simulink model "exp9_"  (R2021b)
settings: Solver=VariableStepAuto  StartTime=0.0  StopTime=100  RelTol=1e-3
undefined symbols (not defined in the file or in its folder): k, k2, k3
libraries: spspowerguiLib x2
settings Model: Creator=amans  LastModifiedBy=amans

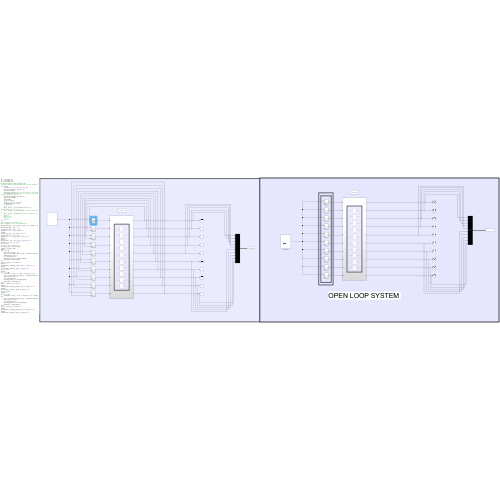
[thumbnail: Simulink's stored preview of the top-level diagram]
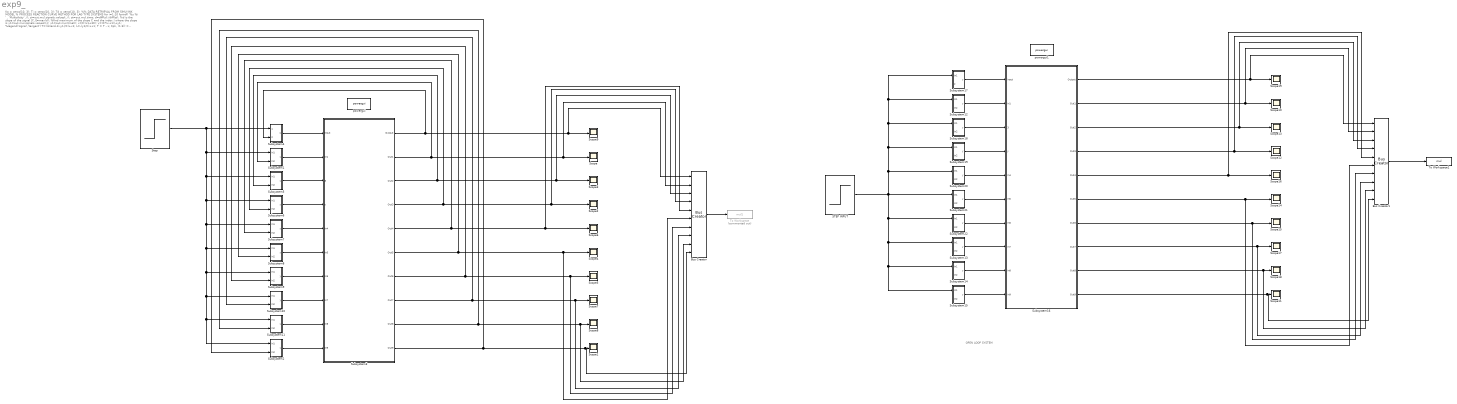
== system exp9_ ==
  note: OPEN LOOP SYSTEM
  note: Kp = zeros(10, 3);
      | Ti = zeros(10, 3);
      | Td = zeros(10, 3);
      | %% DATA RETRIEVAL FROM SIMULINK MODEL
      | % PROCESS REACTION CURVE METHOD FOR LAG TYPE SYSTEMS
      | for i=1:10
      | fprintf( '%s %i\n' , 'Multiplicity' ,i);
      | si=out.mul.signals.values(:,i);
      | st=out.mul.time;
      | d=diff(si)./diff(st); %d is the slope of the signal
      | [C,I]=max(d); %find maximum of the slope C and the index I where the slope is
      | y1=out.mul.signals.values(I,i);
      | x1=out.mul.time(I);
      | x=0:(x1+30);
      | y=(C*(x-x1))+y1;
      | %legend('signal','tangent')
      | T=((si(end-1)-y1)/C)+x1;
      | L=-(y1/C)+x1;
      | T = T - L;
      | Kp(i, (1:3)) = [(T)/L;0.9*T/L;1.2*T/L]; % prooprtional gain for P, Pi, Pid
      | Ti(i, (1:3)) = [-1;L/0.3;2*L]; % time constant for I
      | Td(i, (1:3)) = [0;0;0.5*L]; % time constant for D
      | %hold on
      | %plot(st,si)
      | %plot(x,y);
      | %hold on
      | end
      | %% Dependencies on Multiplicity
      | mul = (1:10); % array for multiplicity
      | scatter(mul,Kp(:, 1)); grid on ; grid minor ; hold on ; % P
      | scatter(mul,Kp(:, 2)); % PI
      | scatter(mul,Kp(:, 3)); % PID
      | legend( 'P' , 'PI' , 'PID' ); hold off ;
      | figure;
      | scatter(mul,Ti(:, 2));hold on ; % PI;
      | scatter(mul,Ti(:, 3)); %PID;
      | legend( 'PI' , 'PID' ); grid on ; grid minor ;
      | hold off ;
      | figure;
      | scatter(mul, Td(:, 3)); grid on ; grid minor ;
      | legend( 'Td vs mul for PID' )
      | %% P CONTROL
      | s = tf( 's' ); H = 1/(s+1.5);
      | settling_Time = zeros(1, 10);
      | oshoot = zeros(1, 10);
      | figure;
      | for i = 1:10
      | controller = Kp(i, 1);
      | cltf = ((controller)*(H^i))/(1 + controller*(H^i));
      | step(cltf); hold on ;
      | A = stepinfo(cltf);
      | settling_Time(i) = A.SettlingTime;
      | oshoot(i) = A.Overshoot;
      | end
      | grid on ; grid minor ; hold off ;
      | figure;
      | scatter(mul, settling_Time); grid on ; grid minor ;
      | figure;
      | scatter(mul, oshoot); grid on ; grid minor ;
      | %% PI control
      | figure;
      | for i = 1:10
      | controller = Kp(i, 2) + Kp(i, 2)/(s*Ti(i, 2));
      | cltf = ((controller)*(H^i))/(1 + controller*(H^i));
      | step(cltf); hold on ;
      | A = stepinfo(cltf);
      | settling_Time(i) = A.SettlingTime;
      | oshoot(i) = A.Overshoot;
      | end
      | grid on ; grid minor ; hold off ;
      | figure;
      | scatter(mul, settling_Time); grid on ; grid minor ;
      | figure;
      | scatter(mul, oshoot); grid on ; grid minor ;
      | %% PID CONTROL
      | figure;
      | for i = 1:10
      | controller = Kp(i, 3)*(1 + 1/(s*Ti(i, 3)) + s*Td(i, 3));
      | cltf = ((controller)*(H^i))/(1 + controller*(H^i));
      | step(cltf); hold on ;
      | A = stepinfo(cltf);
      | settling_Time(i) = A.SettlingTime;
      | oshoot(i) = A.Overshoot;
      | end
      | grid on ; grid minor ; hold off ;
      | figure;
      | scatter(mul, settling_Time); grid on ; grid minor ;
      | figure;
      | scatter(mul, oshoot); grid on ; grid minor ;
  Bus Creator : BusCreator  Inputs=10
  Bus Creator1 : BusCreator  Inputs=10
  STEP INPUT : Step  Time=0  SampleTime=0
  Scope{,1..19} (20 alike) : Scope
  Step : Step  SampleTime=0
  Subsystem1 : Subsystem
  Subsystem10 : Subsystem
  Subsystem11 : Subsystem
  Subsystem12 : Subsystem
  Subsystem13 : Subsystem
  Subsystem14 : Subsystem
  Subsystem15 : Subsystem
  Subsystem16 : Subsystem
  Subsystem17 : Subsystem
  Subsystem18 : Subsystem
  Subsystem19 : Subsystem
  Subsystem2 : Subsystem
  Subsystem20 : Subsystem
  Subsystem21 : Subsystem
  Subsystem22 : Subsystem
  Subsystem3 : Subsystem
  Subsystem4 : Subsystem
  Subsystem5 : Subsystem
  Subsystem6 : Subsystem
  Subsystem7 : Subsystem
  Subsystem8 : Subsystem
  Subsystem9 : Subsystem
  To Workspace : ToWorkspace  Commented=on  VariableName=mul1  SaveFormat=Structure With Time  SampleTime=-1
  To Workspace1 : ToWorkspace  VariableName=mul  SaveFormat=Structure With Time  SampleTime=-1
  powergui : spspowerguiLib/powergui  Priority=1  SimulationMode=Continuous  SampleTime=50e-6  frequency=60  Iterations=50  frequencyindice=60  Pbase=100e6  ErrMax=1e-4  UnitsV=kV  UnitsW=MW  buscounter=0  FunctionMessages=off  echomessages=off  EnableUseOfTLC=off  CurrentSourceSwitches=off  DisableSnubberDevices=off  DisableRonSwitches=off  DisableVfSwitches=off  DisplayEquations=off  AutomaticDiscreteSolvers=off  SolverType=Tustin/Backward Euler (TBE)  Interpol=off  ExternalGateDelay=off  methode=off  Ts=100  x0status=blocks  SPID=on  SwTol=0  HookPort=off  NonlinearTolerance=1e-4  nMaxIteration=100  ContinueOnMaxIteration=off  RestoreLinks=warning  ResistiveCurrentMeasurement=off  Frange=[0:2:500]  Ylog=off  Xlog=on  ShowGrid=off  save=off  variable=ZData  structure=0  ZoomFFT=off  StartTime=0.0  cycles=1  DisplayStyle=1  fundamental=60  FreqAxis=off  MaxFrequency=1000  frequencyindicesteady=1  RmsSteady=1  display=off
  powergui1 : spspowerguiLib/powergui  Priority=1  SimulationMode=Continuous  SampleTime=50e-6  frequency=60  Iterations=50  frequencyindice=60  Pbase=100e6  ErrMax=1e-4  UnitsV=kV  UnitsW=MW  buscounter=0  FunctionMessages=off  echomessages=off  EnableUseOfTLC=off  CurrentSourceSwitches=off  DisableSnubberDevices=off  DisableRonSwitches=off  DisableVfSwitches=off  DisplayEquations=off  AutomaticDiscreteSolvers=off  SolverType=Tustin/Backward Euler (TBE)  Interpol=off  ExternalGateDelay=off  methode=off  Ts=100  x0status=blocks  SPID=on  SwTol=0  HookPort=off  NonlinearTolerance=1e-4  nMaxIteration=100  ContinueOnMaxIteration=off  RestoreLinks=warning  ResistiveCurrentMeasurement=off  Frange=[0:2:500]  Ylog=off  Xlog=on  ShowGrid=off  save=off  variable=ZData  structure=0  ZoomFFT=off  StartTime=0.0  cycles=1  DisplayStyle=1  fundamental=60  FreqAxis=off  MaxFrequency=1000  frequencyindicesteady=1  RmsSteady=1  display=off
  wires:
  Subsystem1/1(y) -> Subsystem3/2(In1)
  Step/1 -> Subsystem9/1(In1), Subsystem10/1(In1), Subsystem2/1(In1), Subsystem11/1(In1), Subsystem8/1(In1), Subsystem7/1(In1), Subsystem6/1(In1), Subsystem5/1(In1), Subsystem1/1(In1), Subsystem4/1(Reference input)
  Subsystem2/1(y) -> Subsystem3/10(In9)
  Subsystem3/10(Out9) -> Bus Creator/10, Scope1/1, Subsystem2/2(In2)
  Subsystem3/2(Out1) -> Subsystem1/2(In2), Scope/1, Bus Creator/2
  Subsystem3/3(Out2) -> Subsystem5/2(In2), Scope3/1, Bus Creator/3
  Subsystem3/5(Out4) -> Subsystem7/2(In2), Scope6/1, Bus Creator/5
  Subsystem3/8(Out7) -> Subsystem10/2(In2), Scope7/1, Bus Creator/8
  Subsystem3/9(Out8) -> Subsystem11/2(In2), Bus Creator/9, Scope8/1
  Subsystem3/1(Output) -> Subsystem4/2(From output), Bus Creator/1, Scope9/1
  Subsystem4/1(To Plant) -> Subsystem3/1(Input)
  Subsystem5/1(y) -> Subsystem3/3(3)
  Subsystem6/1(y) -> Subsystem3/4(y)
  Subsystem7/1(y) -> Subsystem3/5(In4)
  Subsystem8/1(y) -> Subsystem3/6(In5)
  Subsystem3/6(Out5) -> Subsystem8/2(In2), Scope4/1, Bus Creator/6
  Subsystem9/1(y) -> Subsystem3/7(In6)
  Subsystem3/7(Out6) -> Subsystem9/2(In2), Scope5/1, Bus Creator/7
  Subsystem10/1(y) -> Subsystem3/8(In7)
  Subsystem11/1(y) -> Subsystem3/9(In8)
  Bus Creator/1 -> To Workspace/1
  Subsystem3/4(Out3) -> Subsystem6/2(In2), Scope2/1, Bus Creator/4
  Subsystem22/1(y) -> Subsystem16/7(In6)
  Subsystem16/9(Out8) -> Bus Creator1/9, Scope18/1
  Subsystem17/1(y) -> Subsystem16/1(Input)
  Subsystem16/4(Out3) -> Scope12/1, Bus Creator1/4
  Subsystem16/1(Output) -> Bus Creator1/1, Scope19/1
  Subsystem16/7(Out6) -> Scope15/1, Bus Creator1/7
  Subsystem20/1(y) -> Subsystem16/5(In4)
  Subsystem18/1(y) -> Subsystem16/3(3)
  Subsystem12/1(y) -> Subsystem16/2(In1)
  Subsystem16/5(Out4) -> Scope16/1, Bus Creator1/5
  Subsystem15/1(y) -> Subsystem16/10(In9)
  Bus Creator1/1 -> To Workspace1/1
  Subsystem19/1(y) -> Subsystem16/4(y)
  Subsystem21/1(y) -> Subsystem16/6(In5)
  Subsystem16/10(Out9) -> Bus Creator1/10, Scope11/1
  Subsystem16/2(Out1) -> Scope10/1, Bus Creator1/2
  Subsystem16/3(Out2) -> Scope13/1, Bus Creator1/3
  Subsystem13/1(y) -> Subsystem16/8(In7)
  Subsystem14/1(y) -> Subsystem16/9(In8)
  Subsystem16/6(Out5) -> Scope14/1, Bus Creator1/6
  Subsystem16/8(Out7) -> Scope17/1, Bus Creator1/8
  STEP INPUT/1 -> Subsystem17/1(In1), Subsystem12/1(In1), Subsystem18/1(In1), Subsystem19/1(In1), Subsystem20/1(In1), Subsystem22/1(In1), Subsystem13/1(In1), Subsystem15/1(In1), Subsystem14/1(In1), Subsystem21/1(In1)

== system exp9_/Subsystem1 ==
  In1 : Inport
  In2 : Inport  Port=2
  Sum : Sum  Inputs=|+-
  y : Outport
  wires:
  In1/1 -> Sum/1
  In2/1 -> Sum/2
  Sum/1 -> y/1

== system exp9_/Subsystem10 ==
  In1 : Inport
  In2 : Inport  Port=2
  Sum : Sum  Inputs=|+-
  y : Outport
  wires:
  In1/1 -> Sum/1
  In2/1 -> Sum/2
  Sum/1 -> y/1

== system exp9_/Subsystem11 ==
  In1 : Inport
  In2 : Inport  Port=2
  Sum : Sum  Inputs=|+-
  y : Outport
  wires:
  In1/1 -> Sum/1
  In2/1 -> Sum/2
  Sum/1 -> y/1

== system exp9_/Subsystem12 ==
  In1 : Inport
  In2 : Inport  Port=2
  Sum : Sum  Inputs=|+-
  y : Outport
  wires:
  In1/1 -> Sum/1
  In2/1 -> Sum/2
  Sum/1 -> y/1

== system exp9_/Subsystem13 ==
  In1 : Inport
  In2 : Inport  Port=2
  Sum : Sum  Inputs=|+-
  y : Outport
  wires:
  In1/1 -> Sum/1
  In2/1 -> Sum/2
  Sum/1 -> y/1

== system exp9_/Subsystem14 ==
  In1 : Inport
  In2 : Inport  Port=2
  Sum : Sum  Inputs=|+-
  y : Outport
  wires:
  In1/1 -> Sum/1
  In2/1 -> Sum/2
  Sum/1 -> y/1

== system exp9_/Subsystem15 ==
  In1 : Inport
  In2 : Inport  Port=2
  Sum : Sum  Inputs=|+-
  y : Outport
  wires:
  In1/1 -> Sum/1
  In2/1 -> Sum/2
  Sum/1 -> y/1

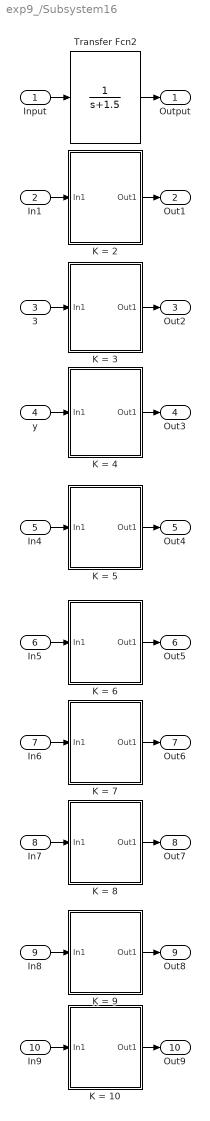
== system exp9_/Subsystem16 ==
  Input : Inport
  In1 : Inport  Port=2
  3 : Inport  Port=3
  y : Inport  Port=4
  In4 : Inport  Port=5
  In5 : Inport  Port=6
  In6 : Inport  Port=7
  In7 : Inport  Port=8
  In8 : Inport  Port=9
  In9 : Inport  Port=10
  K = 10 : Subsystem
  K = 2 : Subsystem
  K = 3 : Subsystem
  K = 4 : Subsystem
  K = 5 : Subsystem
  K = 6 : Subsystem
  K = 7 : Subsystem
  K = 8 : Subsystem
  K = 9 : Subsystem
  Transfer Fcn2 : TransferFcn  Denominator=[1 1.5]
  Output : Outport
  Out1 : Outport  Port=2
  Out2 : Outport  Port=3
  Out3 : Outport  Port=4
  Out4 : Outport  Port=5
  Out5 : Outport  Port=6
  Out6 : Outport  Port=7
  Out7 : Outport  Port=8
  Out8 : Outport  Port=9
  Out9 : Outport  Port=10
  wires:
  K = 8/1(Out1) -> Out7/1
  3/1 -> K = 3/1(In1)
  In9/1 -> K = 10/1(In1)
  K = 6/1(Out1) -> Out5/1
  K = 3/1(Out1) -> Out2/1
  K = 9/1(Out1) -> Out8/1
  K = 2/1(Out1) -> Out1/1
  In8/1 -> K = 9/1(In1)
  K = 10/1(Out1) -> Out9/1
  In6/1 -> K = 7/1(In1)
  In4/1 -> K = 5/1(In1)
  In7/1 -> K = 8/1(In1)
  K = 4/1(Out1) -> Out3/1
  y/1 -> K = 4/1(In1)
  K = 7/1(Out1) -> Out6/1
  In5/1 -> K = 6/1(In1)
  In1/1 -> K = 2/1(In1)
  K = 5/1(Out1) -> Out4/1
  Input/1 -> Transfer Fcn2/1
  Transfer Fcn2/1 -> Output/1

== system exp9_/Subsystem17 ==
  In1 : Inport
  Output : Inport  Port=2
  Sum : Sum  Inputs=|+-
  y : Outport
  wires:
  In1/1 -> Sum/1
  Output/1 -> Sum/2
  Sum/1 -> y/1

== system exp9_/Subsystem18 ==
  In1 : Inport
  In2 : Inport  Port=2
  Sum : Sum  Inputs=|+-
  y : Outport
  wires:
  In1/1 -> Sum/1
  In2/1 -> Sum/2
  Sum/1 -> y/1

== system exp9_/Subsystem19 ==
  In1 : Inport
  In2 : Inport  Port=2
  Sum : Sum  Inputs=|+-
  y : Outport
  wires:
  In1/1 -> Sum/1
  In2/1 -> Sum/2
  Sum/1 -> y/1

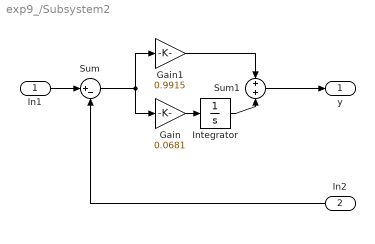
== system exp9_/Subsystem2 ==
  In1 : Inport
  In2 : Inport  Port=2
  Gain : Gain  Gain=0.0681
  Gain1 : Gain  Gain=0.9915
  Integrator : Integrator
  Sum : Sum  Inputs=|+-
  Sum1 : Sum  Inputs=+|+
  y : Outport
  wires:
  In1/1 -> Sum/1
  In2/1 -> Sum/2
  Gain/1 -> Integrator/1
  Sum/1 -> Gain1/1, Gain/1
  Sum1/1 -> y/1
  Integrator/1 -> Sum1/2
  Gain1/1 -> Sum1/1

== system exp9_/Subsystem20 ==
  In1 : Inport
  In2 : Inport  Port=2
  Sum : Sum  Inputs=|+-
  y : Outport
  wires:
  In1/1 -> Sum/1
  In2/1 -> Sum/2
  Sum/1 -> y/1

== system exp9_/Subsystem21 ==
  In1 : Inport
  In2 : Inport  Port=2
  Sum : Sum  Inputs=|+-
  y : Outport
  wires:
  In1/1 -> Sum/1
  In2/1 -> Sum/2
  Sum/1 -> y/1

== system exp9_/Subsystem22 ==
  In1 : Inport
  In2 : Inport  Port=2
  Sum : Sum  Inputs=|+-
  y : Outport
  wires:
  In1/1 -> Sum/1
  In2/1 -> Sum/2
  Sum/1 -> y/1

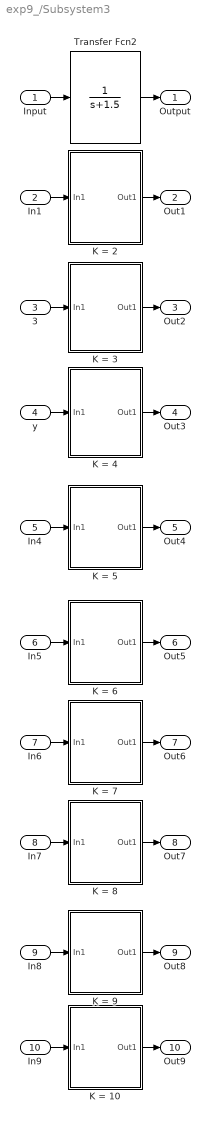
== system exp9_/Subsystem3 ==
  Input : Inport
  In1 : Inport  Port=2
  3 : Inport  Port=3
  y : Inport  Port=4
  In4 : Inport  Port=5
  In5 : Inport  Port=6
  In6 : Inport  Port=7
  In7 : Inport  Port=8
  In8 : Inport  Port=9
  In9 : Inport  Port=10
  K = 10 : Subsystem
  K = 2 : Subsystem
  K = 3 : Subsystem
  K = 4 : Subsystem
  K = 5 : Subsystem
  K = 6 : Subsystem
  K = 7 : Subsystem
  K = 8 : Subsystem
  K = 9 : Subsystem
  Transfer Fcn2 : TransferFcn  Denominator=[1 1.5]
  Output : Outport
  Out1 : Outport  Port=2
  Out2 : Outport  Port=3
  Out3 : Outport  Port=4
  Out4 : Outport  Port=5
  Out5 : Outport  Port=6
  Out6 : Outport  Port=7
  Out7 : Outport  Port=8
  Out8 : Outport  Port=9
  Out9 : Outport  Port=10
  wires:
  K = 8/1(Out1) -> Out7/1
  3/1 -> K = 3/1(In1)
  In9/1 -> K = 10/1(In1)
  K = 6/1(Out1) -> Out5/1
  K = 3/1(Out1) -> Out2/1
  K = 9/1(Out1) -> Out8/1
  K = 2/1(Out1) -> Out1/1
  In8/1 -> K = 9/1(In1)
  K = 10/1(Out1) -> Out9/1
  In6/1 -> K = 7/1(In1)
  In4/1 -> K = 5/1(In1)
  In7/1 -> K = 8/1(In1)
  K = 4/1(Out1) -> Out3/1
  y/1 -> K = 4/1(In1)
  K = 7/1(Out1) -> Out6/1
  In5/1 -> K = 6/1(In1)
  In1/1 -> K = 2/1(In1)
  K = 5/1(Out1) -> Out4/1
  Input/1 -> Transfer Fcn2/1
  Transfer Fcn2/1 -> Output/1

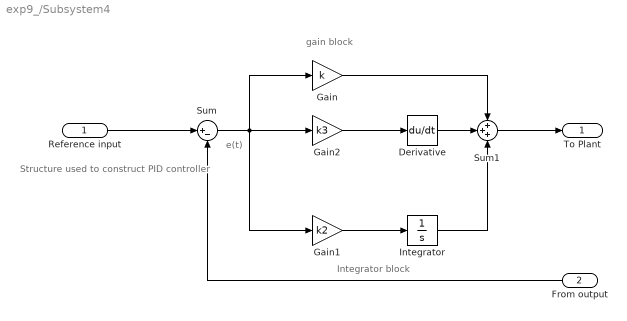
== system exp9_/Subsystem4 ==
  note: Integrator block
  note: Structure used to construct PID controller
  note: gain block
  note: e(t)
  Reference input : Inport
  From output : Inport  Port=2
  Derivative : Derivative
  Gain : Gain  Gain=k
  Gain1 : Gain  Gain=k2
  Gain2 : Gain  Gain=k3
  Integrator : Integrator
  Sum : Sum  Inputs=|+-
  Sum1 : Sum  Inputs=+++
  To Plant : Outport
  wires:
  Reference input/1 -> Sum/1
  From output/1 -> Sum/2
  Sum/1 -> Gain2/1, Gain/1, Gain1/1
  Integrator/1 -> Sum1/3
  Sum1/1 -> To Plant/1
  Gain/1 -> Sum1/1
  Gain1/1 -> Integrator/1
  Derivative/1 -> Sum1/2
  Gain2/1 -> Derivative/1

== system exp9_/Subsystem5 ==
  In1 : Inport
  In2 : Inport  Port=2
  Sum : Sum  Inputs=|+-
  y : Outport
  wires:
  In1/1 -> Sum/1
  In2/1 -> Sum/2
  Sum/1 -> y/1

== system exp9_/Subsystem6 ==
  In1 : Inport
  In2 : Inport  Port=2
  Sum : Sum  Inputs=|+-
  y : Outport
  wires:
  In1/1 -> Sum/1
  In2/1 -> Sum/2
  Sum/1 -> y/1

== system exp9_/Subsystem7 ==
  In1 : Inport
  In2 : Inport  Port=2
  Sum : Sum  Inputs=|+-
  y : Outport
  wires:
  In1/1 -> Sum/1
  In2/1 -> Sum/2
  Sum/1 -> y/1

== system exp9_/Subsystem8 ==
  In1 : Inport
  In2 : Inport  Port=2
  Sum : Sum  Inputs=|+-
  y : Outport
  wires:
  In1/1 -> Sum/1
  In2/1 -> Sum/2
  Sum/1 -> y/1

== system exp9_/Subsystem9 ==
  In1 : Inport
  In2 : Inport  Port=2
  Sum : Sum  Inputs=|+-
  y : Outport
  wires:
  In1/1 -> Sum/1
  In2/1 -> Sum/2
  Sum/1 -> y/1

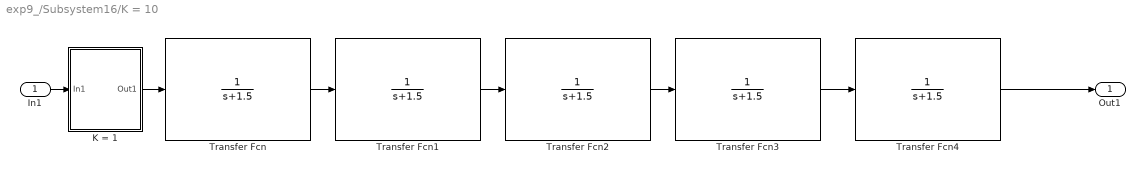
== system exp9_/Subsystem16/K = 10 ==
  In1 : Inport
  K = 1 : Subsystem
  Transfer Fcn{,1..4} (5 alike) : TransferFcn  Denominator=[1 1.5]
  Out1 : Outport
  wires:
  K = 1/1(Out1) -> Transfer Fcn/1
  In1/1 -> K = 1/1(In1)
  Transfer Fcn/1 -> Transfer Fcn1/1
  Transfer Fcn1/1 -> Transfer Fcn2/1
  Transfer Fcn2/1 -> Transfer Fcn3/1
  Transfer Fcn3/1 -> Transfer Fcn4/1
  Transfer Fcn4/1 -> Out1/1

== system exp9_/Subsystem16/K = 2 ==
  In1 : Inport
  Transfer Fcn2 : TransferFcn  Denominator=[1 1.5]
  Transfer Fcn3 : TransferFcn  Denominator=[1 1.5]
  Out1 : Outport
  wires:
  Transfer Fcn2/1 -> Transfer Fcn3/1
  In1/1 -> Transfer Fcn2/1
  Transfer Fcn3/1 -> Out1/1

== system exp9_/Subsystem16/K = 3 ==
  In1 : Inport
  K = 1 : Subsystem
  Transfer Fcn2 : TransferFcn  Denominator=[1 1.5]
  Out1 : Outport
  wires:
  K = 1/1(Out1) -> Transfer Fcn2/1
  Transfer Fcn2/1 -> Out1/1
  In1/1 -> K = 1/1(In1)

== system exp9_/Subsystem16/K = 4 ==
  In1 : Inport
  K = 1 : Subsystem
  Transfer Fcn2 : TransferFcn  Denominator=[1 1.5]
  Out1 : Outport
  wires:
  K = 1/1(Out1) -> Transfer Fcn2/1
  Transfer Fcn2/1 -> Out1/1
  In1/1 -> K = 1/1(In1)

== system exp9_/Subsystem16/K = 5 ==
  In1 : Inport
  K = 1 : Subsystem
  Transfer Fcn : TransferFcn  Denominator=[1 1.5]
  Out1 : Outport
  wires:
  K = 1/1(Out1) -> Transfer Fcn/1
  In1/1 -> K = 1/1(In1)
  Transfer Fcn/1 -> Out1/1

== system exp9_/Subsystem16/K = 6 ==
  In1 : Inport
  K = 1 : Subsystem
  Transfer Fcn : TransferFcn  Denominator=[1 1.5]
  Out1 : Outport
  wires:
  Transfer Fcn/1 -> Out1/1
  K = 1/1(Out1) -> Transfer Fcn/1
  In1/1 -> K = 1/1(In1)

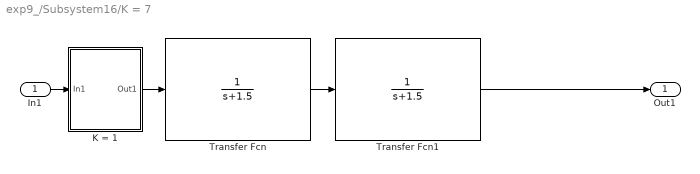
== system exp9_/Subsystem16/K = 7 ==
  In1 : Inport
  K = 1 : Subsystem
  Transfer Fcn : TransferFcn  Denominator=[1 1.5]
  Transfer Fcn1 : TransferFcn  Denominator=[1 1.5]
  Out1 : Outport
  wires:
  K = 1/1(Out1) -> Transfer Fcn/1
  In1/1 -> K = 1/1(In1)
  Transfer Fcn/1 -> Transfer Fcn1/1
  Transfer Fcn1/1 -> Out1/1

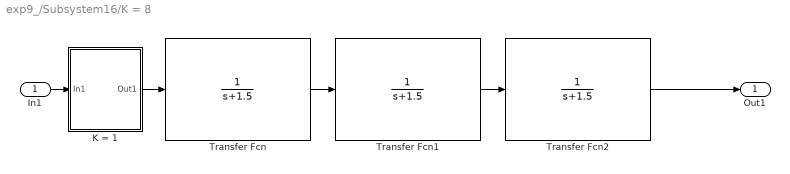
== system exp9_/Subsystem16/K = 8 ==
  In1 : Inport
  K = 1 : Subsystem
  Transfer Fcn : TransferFcn  Denominator=[1 1.5]
  Transfer Fcn1 : TransferFcn  Denominator=[1 1.5]
  Transfer Fcn2 : TransferFcn  Denominator=[1 1.5]
  Out1 : Outport
  wires:
  K = 1/1(Out1) -> Transfer Fcn/1
  In1/1 -> K = 1/1(In1)
  Transfer Fcn/1 -> Transfer Fcn1/1
  Transfer Fcn1/1 -> Transfer Fcn2/1
  Transfer Fcn2/1 -> Out1/1

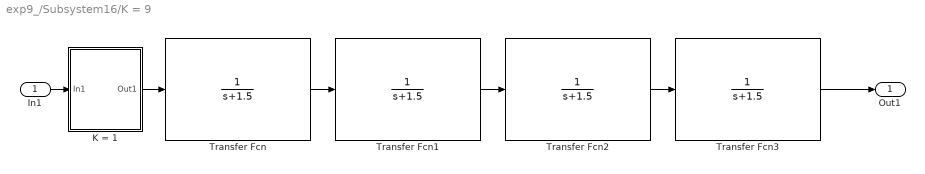
== system exp9_/Subsystem16/K = 9 ==
  In1 : Inport
  K = 1 : Subsystem
  Transfer Fcn{,1..3} (4 alike) : TransferFcn  Denominator=[1 1.5]
  Out1 : Outport
  wires:
  K = 1/1(Out1) -> Transfer Fcn/1
  In1/1 -> K = 1/1(In1)
  Transfer Fcn/1 -> Transfer Fcn1/1
  Transfer Fcn1/1 -> Transfer Fcn2/1
  Transfer Fcn2/1 -> Transfer Fcn3/1
  Transfer Fcn3/1 -> Out1/1

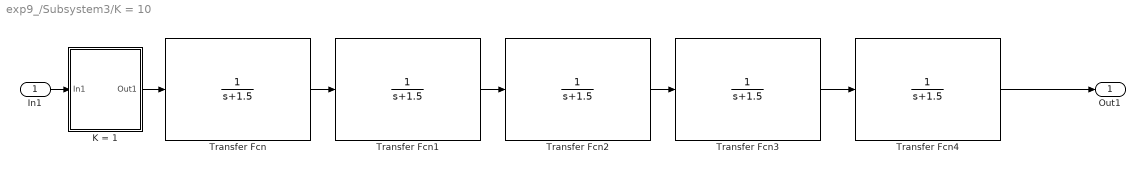
== system exp9_/Subsystem3/K = 10 ==
  In1 : Inport
  K = 1 : Subsystem
  Transfer Fcn{,1..4} (5 alike) : TransferFcn  Denominator=[1 1.5]
  Out1 : Outport
  wires:
  K = 1/1(Out1) -> Transfer Fcn/1
  In1/1 -> K = 1/1(In1)
  Transfer Fcn/1 -> Transfer Fcn1/1
  Transfer Fcn1/1 -> Transfer Fcn2/1
  Transfer Fcn2/1 -> Transfer Fcn3/1
  Transfer Fcn3/1 -> Transfer Fcn4/1
  Transfer Fcn4/1 -> Out1/1

== system exp9_/Subsystem3/K = 2 ==
  In1 : Inport
  Transfer Fcn2 : TransferFcn  Denominator=[1 1.5]
  Transfer Fcn3 : TransferFcn  Denominator=[1 1.5]
  Out1 : Outport
  wires:
  Transfer Fcn2/1 -> Transfer Fcn3/1
  In1/1 -> Transfer Fcn2/1
  Transfer Fcn3/1 -> Out1/1

== system exp9_/Subsystem3/K = 3 ==
  In1 : Inport
  K = 1 : Subsystem
  Transfer Fcn2 : TransferFcn  Denominator=[1 1.5]
  Out1 : Outport
  wires:
  K = 1/1(Out1) -> Transfer Fcn2/1
  Transfer Fcn2/1 -> Out1/1
  In1/1 -> K = 1/1(In1)

== system exp9_/Subsystem3/K = 4 ==
  In1 : Inport
  K = 1 : Subsystem
  Transfer Fcn2 : TransferFcn  Denominator=[1 1.5]
  Out1 : Outport
  wires:
  K = 1/1(Out1) -> Transfer Fcn2/1
  Transfer Fcn2/1 -> Out1/1
  In1/1 -> K = 1/1(In1)

== system exp9_/Subsystem3/K = 5 ==
  In1 : Inport
  K = 1 : Subsystem
  Transfer Fcn : TransferFcn  Denominator=[1 1.5]
  Out1 : Outport
  wires:
  K = 1/1(Out1) -> Transfer Fcn/1
  In1/1 -> K = 1/1(In1)
  Transfer Fcn/1 -> Out1/1

== system exp9_/Subsystem3/K = 6 ==
  In1 : Inport
  K = 1 : Subsystem
  Transfer Fcn : TransferFcn  Denominator=[1 1.5]
  Out1 : Outport
  wires:
  Transfer Fcn/1 -> Out1/1
  K = 1/1(Out1) -> Transfer Fcn/1
  In1/1 -> K = 1/1(In1)

== system exp9_/Subsystem3/K = 7 ==
  In1 : Inport
  K = 1 : Subsystem
  Transfer Fcn : TransferFcn  Denominator=[1 1.5]
  Transfer Fcn1 : TransferFcn  Denominator=[1 1.5]
  Out1 : Outport
  wires:
  K = 1/1(Out1) -> Transfer Fcn/1
  In1/1 -> K = 1/1(In1)
  Transfer Fcn/1 -> Transfer Fcn1/1
  Transfer Fcn1/1 -> Out1/1

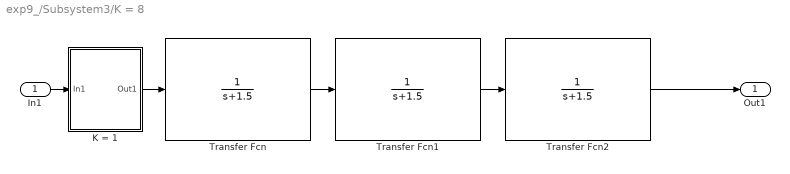
== system exp9_/Subsystem3/K = 8 ==
  In1 : Inport
  K = 1 : Subsystem
  Transfer Fcn : TransferFcn  Denominator=[1 1.5]
  Transfer Fcn1 : TransferFcn  Denominator=[1 1.5]
  Transfer Fcn2 : TransferFcn  Denominator=[1 1.5]
  Out1 : Outport
  wires:
  K = 1/1(Out1) -> Transfer Fcn/1
  In1/1 -> K = 1/1(In1)
  Transfer Fcn/1 -> Transfer Fcn1/1
  Transfer Fcn1/1 -> Transfer Fcn2/1
  Transfer Fcn2/1 -> Out1/1

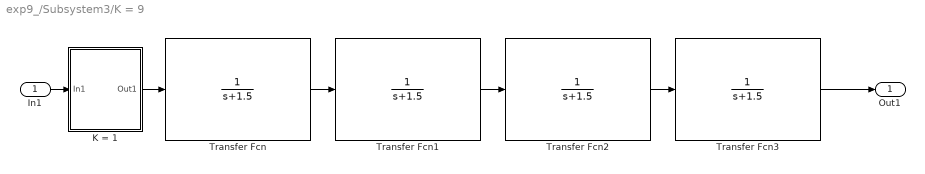
== system exp9_/Subsystem3/K = 9 ==
  In1 : Inport
  K = 1 : Subsystem
  Transfer Fcn{,1..3} (4 alike) : TransferFcn  Denominator=[1 1.5]
  Out1 : Outport
  wires:
  K = 1/1(Out1) -> Transfer Fcn/1
  In1/1 -> K = 1/1(In1)
  Transfer Fcn/1 -> Transfer Fcn1/1
  Transfer Fcn1/1 -> Transfer Fcn2/1
  Transfer Fcn2/1 -> Transfer Fcn3/1
  Transfer Fcn3/1 -> Out1/1

== system exp9_/Subsystem16/K = 10/K = 1 ==
  In1 : Inport
  K = 1 : Subsystem
  Transfer Fcn : TransferFcn  Denominator=[1 1.5]
  Out1 : Outport
  wires:
  K = 1/1(Out1) -> Transfer Fcn/1
  In1/1 -> K = 1/1(In1)
  Transfer Fcn/1 -> Out1/1

== system exp9_/Subsystem16/K = 3/K = 1 ==
  In1 : Inport
  Transfer Fcn2 : TransferFcn  Denominator=[1 1.5]
  Transfer Fcn3 : TransferFcn  Denominator=[1 1.5]
  Out1 : Outport
  wires:
  Transfer Fcn2/1 -> Transfer Fcn3/1
  In1/1 -> Transfer Fcn2/1
  Transfer Fcn3/1 -> Out1/1

== system exp9_/Subsystem16/K = 4/K = 1 ==
  In1 : Inport
  Transfer Fcn2 : TransferFcn  Denominator=[1 1.5]
  Transfer Fcn3 : TransferFcn  Denominator=[1 1.5]
  Out1 : Outport
  wires:
  Transfer Fcn2/1 -> Transfer Fcn3/1
  In1/1 -> Transfer Fcn2/1
  Transfer Fcn3/1 -> Out1/1

== system exp9_/Subsystem16/K = 5/K = 1 ==
  In1 : Inport
  K = 1 : Subsystem
  Transfer Fcn2 : TransferFcn  Denominator=[1 1.5]
  Out1 : Outport
  wires:
  K = 1/1(Out1) -> Transfer Fcn2/1
  Transfer Fcn2/1 -> Out1/1
  In1/1 -> K = 1/1(In1)

== system exp9_/Subsystem16/K = 6/K = 1 ==
  In1 : Inport
  K = 1 : Subsystem
  Transfer Fcn : TransferFcn  Denominator=[1 1.5]
  Out1 : Outport
  wires:
  K = 1/1(Out1) -> Transfer Fcn/1
  In1/1 -> K = 1/1(In1)
  Transfer Fcn/1 -> Out1/1

== system exp9_/Subsystem16/K = 7/K = 1 ==
  In1 : Inport
  K = 1 : Subsystem
  Transfer Fcn : TransferFcn  Denominator=[1 1.5]
  Out1 : Outport
  wires:
  K = 1/1(Out1) -> Transfer Fcn/1
  In1/1 -> K = 1/1(In1)
  Transfer Fcn/1 -> Out1/1

== system exp9_/Subsystem16/K = 8/K = 1 ==
  In1 : Inport
  K = 1 : Subsystem
  Transfer Fcn : TransferFcn  Denominator=[1 1.5]
  Out1 : Outport
  wires:
  K = 1/1(Out1) -> Transfer Fcn/1
  In1/1 -> K = 1/1(In1)
  Transfer Fcn/1 -> Out1/1

== system exp9_/Subsystem16/K = 9/K = 1 ==
  In1 : Inport
  K = 1 : Subsystem
  Transfer Fcn : TransferFcn  Denominator=[1 1.5]
  Out1 : Outport
  wires:
  K = 1/1(Out1) -> Transfer Fcn/1
  In1/1 -> K = 1/1(In1)
  Transfer Fcn/1 -> Out1/1

== system exp9_/Subsystem3/K = 10/K = 1 ==
  In1 : Inport
  K = 1 : Subsystem
  Transfer Fcn : TransferFcn  Denominator=[1 1.5]
  Out1 : Outport
  wires:
  K = 1/1(Out1) -> Transfer Fcn/1
  In1/1 -> K = 1/1(In1)
  Transfer Fcn/1 -> Out1/1

== system exp9_/Subsystem3/K = 3/K = 1 ==
  In1 : Inport
  Transfer Fcn2 : TransferFcn  Denominator=[1 1.5]
  Transfer Fcn3 : TransferFcn  Denominator=[1 1.5]
  Out1 : Outport
  wires:
  Transfer Fcn2/1 -> Transfer Fcn3/1
  In1/1 -> Transfer Fcn2/1
  Transfer Fcn3/1 -> Out1/1

== system exp9_/Subsystem3/K = 4/K = 1 ==
  In1 : Inport
  Transfer Fcn2 : TransferFcn  Denominator=[1 1.5]
  Transfer Fcn3 : TransferFcn  Denominator=[1 1.5]
  Out1 : Outport
  wires:
  Transfer Fcn2/1 -> Transfer Fcn3/1
  In1/1 -> Transfer Fcn2/1
  Transfer Fcn3/1 -> Out1/1

== system exp9_/Subsystem3/K = 5/K = 1 ==
  In1 : Inport
  K = 1 : Subsystem
  Transfer Fcn2 : TransferFcn  Denominator=[1 1.5]
  Out1 : Outport
  wires:
  K = 1/1(Out1) -> Transfer Fcn2/1
  Transfer Fcn2/1 -> Out1/1
  In1/1 -> K = 1/1(In1)

== system exp9_/Subsystem3/K = 6/K = 1 ==
  In1 : Inport
  K = 1 : Subsystem
  Transfer Fcn : TransferFcn  Denominator=[1 1.5]
  Out1 : Outport
  wires:
  K = 1/1(Out1) -> Transfer Fcn/1
  In1/1 -> K = 1/1(In1)
  Transfer Fcn/1 -> Out1/1

== system exp9_/Subsystem3/K = 7/K = 1 ==
  In1 : Inport
  K = 1 : Subsystem
  Transfer Fcn : TransferFcn  Denominator=[1 1.5]
  Out1 : Outport
  wires:
  K = 1/1(Out1) -> Transfer Fcn/1
  In1/1 -> K = 1/1(In1)
  Transfer Fcn/1 -> Out1/1

== system exp9_/Subsystem3/K = 8/K = 1 ==
  In1 : Inport
  K = 1 : Subsystem
  Transfer Fcn : TransferFcn  Denominator=[1 1.5]
  Out1 : Outport
  wires:
  K = 1/1(Out1) -> Transfer Fcn/1
  In1/1 -> K = 1/1(In1)
  Transfer Fcn/1 -> Out1/1

== system exp9_/Subsystem3/K = 9/K = 1 ==
  In1 : Inport
  K = 1 : Subsystem
  Transfer Fcn : TransferFcn  Denominator=[1 1.5]
  Out1 : Outport
  wires:
  K = 1/1(Out1) -> Transfer Fcn/1
  In1/1 -> K = 1/1(In1)
  Transfer Fcn/1 -> Out1/1

== system exp9_/Subsystem16/K = 10/K = 1/K = 1 ==
  In1 : Inport
  K = 1 : Subsystem
  Transfer Fcn2 : TransferFcn  Denominator=[1 1.5]
  Out1 : Outport
  wires:
  K = 1/1(Out1) -> Transfer Fcn2/1
  Transfer Fcn2/1 -> Out1/1
  In1/1 -> K = 1/1(In1)

== system exp9_/Subsystem16/K = 5/K = 1/K = 1 ==
  In1 : Inport
  Transfer Fcn2 : TransferFcn  Denominator=[1 1.5]
  Transfer Fcn3 : TransferFcn  Denominator=[1 1.5]
  Out1 : Outport
  wires:
  Transfer Fcn2/1 -> Transfer Fcn3/1
  In1/1 -> Transfer Fcn2/1
  Transfer Fcn3/1 -> Out1/1

== system exp9_/Subsystem16/K = 6/K = 1/K = 1 ==
  In1 : Inport
  K = 1 : Subsystem
  Transfer Fcn2 : TransferFcn  Denominator=[1 1.5]
  Out1 : Outport
  wires:
  K = 1/1(Out1) -> Transfer Fcn2/1
  Transfer Fcn2/1 -> Out1/1
  In1/1 -> K = 1/1(In1)

== system exp9_/Subsystem16/K = 7/K = 1/K = 1 ==
  In1 : Inport
  K = 1 : Subsystem
  Transfer Fcn2 : TransferFcn  Denominator=[1 1.5]
  Out1 : Outport
  wires:
  K = 1/1(Out1) -> Transfer Fcn2/1
  Transfer Fcn2/1 -> Out1/1
  In1/1 -> K = 1/1(In1)

== system exp9_/Subsystem16/K = 8/K = 1/K = 1 ==
  In1 : Inport
  K = 1 : Subsystem
  Transfer Fcn2 : TransferFcn  Denominator=[1 1.5]
  Out1 : Outport
  wires:
  K = 1/1(Out1) -> Transfer Fcn2/1
  Transfer Fcn2/1 -> Out1/1
  In1/1 -> K = 1/1(In1)

== system exp9_/Subsystem16/K = 9/K = 1/K = 1 ==
  In1 : Inport
  K = 1 : Subsystem
  Transfer Fcn2 : TransferFcn  Denominator=[1 1.5]
  Out1 : Outport
  wires:
  K = 1/1(Out1) -> Transfer Fcn2/1
  Transfer Fcn2/1 -> Out1/1
  In1/1 -> K = 1/1(In1)

== system exp9_/Subsystem3/K = 10/K = 1/K = 1 ==
  In1 : Inport
  K = 1 : Subsystem
  Transfer Fcn2 : TransferFcn  Denominator=[1 1.5]
  Out1 : Outport
  wires:
  K = 1/1(Out1) -> Transfer Fcn2/1
  Transfer Fcn2/1 -> Out1/1
  In1/1 -> K = 1/1(In1)

== system exp9_/Subsystem3/K = 5/K = 1/K = 1 ==
  In1 : Inport
  Transfer Fcn2 : TransferFcn  Denominator=[1 1.5]
  Transfer Fcn3 : TransferFcn  Denominator=[1 1.5]
  Out1 : Outport
  wires:
  Transfer Fcn2/1 -> Transfer Fcn3/1
  In1/1 -> Transfer Fcn2/1
  Transfer Fcn3/1 -> Out1/1

== system exp9_/Subsystem3/K = 6/K = 1/K = 1 ==
  In1 : Inport
  K = 1 : Subsystem
  Transfer Fcn2 : TransferFcn  Denominator=[1 1.5]
  Out1 : Outport
  wires:
  K = 1/1(Out1) -> Transfer Fcn2/1
  Transfer Fcn2/1 -> Out1/1
  In1/1 -> K = 1/1(In1)

== system exp9_/Subsystem3/K = 7/K = 1/K = 1 ==
  In1 : Inport
  K = 1 : Subsystem
  Transfer Fcn2 : TransferFcn  Denominator=[1 1.5]
  Out1 : Outport
  wires:
  K = 1/1(Out1) -> Transfer Fcn2/1
  Transfer Fcn2/1 -> Out1/1
  In1/1 -> K = 1/1(In1)

== system exp9_/Subsystem3/K = 8/K = 1/K = 1 ==
  In1 : Inport
  K = 1 : Subsystem
  Transfer Fcn2 : TransferFcn  Denominator=[1 1.5]
  Out1 : Outport
  wires:
  K = 1/1(Out1) -> Transfer Fcn2/1
  Transfer Fcn2/1 -> Out1/1
  In1/1 -> K = 1/1(In1)

== system exp9_/Subsystem3/K = 9/K = 1/K = 1 ==
  In1 : Inport
  K = 1 : Subsystem
  Transfer Fcn2 : TransferFcn  Denominator=[1 1.5]
  Out1 : Outport
  wires:
  K = 1/1(Out1) -> Transfer Fcn2/1
  Transfer Fcn2/1 -> Out1/1
  In1/1 -> K = 1/1(In1)

== system exp9_/Subsystem16/K = 10/K = 1/K = 1/K = 1 ==
  In1 : Inport
  Transfer Fcn2 : TransferFcn  Denominator=[1 1.5]
  Transfer Fcn3 : TransferFcn  Denominator=[1 1.5]
  Out1 : Outport
  wires:
  Transfer Fcn2/1 -> Transfer Fcn3/1
  In1/1 -> Transfer Fcn2/1
  Transfer Fcn3/1 -> Out1/1

== system exp9_/Subsystem16/K = 6/K = 1/K = 1/K = 1 ==
  In1 : Inport
  Transfer Fcn2 : TransferFcn  Denominator=[1 1.5]
  Transfer Fcn3 : TransferFcn  Denominator=[1 1.5]
  Out1 : Outport
  wires:
  Transfer Fcn2/1 -> Transfer Fcn3/1
  In1/1 -> Transfer Fcn2/1
  Transfer Fcn3/1 -> Out1/1

== system exp9_/Subsystem16/K = 7/K = 1/K = 1/K = 1 ==
  In1 : Inport
  Transfer Fcn2 : TransferFcn  Denominator=[1 1.5]
  Transfer Fcn3 : TransferFcn  Denominator=[1 1.5]
  Out1 : Outport
  wires:
  Transfer Fcn2/1 -> Transfer Fcn3/1
  In1/1 -> Transfer Fcn2/1
  Transfer Fcn3/1 -> Out1/1

== system exp9_/Subsystem16/K = 8/K = 1/K = 1/K = 1 ==
  In1 : Inport
  Transfer Fcn2 : TransferFcn  Denominator=[1 1.5]
  Transfer Fcn3 : TransferFcn  Denominator=[1 1.5]
  Out1 : Outport
  wires:
  Transfer Fcn2/1 -> Transfer Fcn3/1
  In1/1 -> Transfer Fcn2/1
  Transfer Fcn3/1 -> Out1/1

== system exp9_/Subsystem16/K = 9/K = 1/K = 1/K = 1 ==
  In1 : Inport
  Transfer Fcn2 : TransferFcn  Denominator=[1 1.5]
  Transfer Fcn3 : TransferFcn  Denominator=[1 1.5]
  Out1 : Outport
  wires:
  Transfer Fcn2/1 -> Transfer Fcn3/1
  In1/1 -> Transfer Fcn2/1
  Transfer Fcn3/1 -> Out1/1

== system exp9_/Subsystem3/K = 10/K = 1/K = 1/K = 1 ==
  In1 : Inport
  Transfer Fcn2 : TransferFcn  Denominator=[1 1.5]
  Transfer Fcn3 : TransferFcn  Denominator=[1 1.5]
  Out1 : Outport
  wires:
  Transfer Fcn2/1 -> Transfer Fcn3/1
  In1/1 -> Transfer Fcn2/1
  Transfer Fcn3/1 -> Out1/1

== system exp9_/Subsystem3/K = 6/K = 1/K = 1/K = 1 ==
  In1 : Inport
  Transfer Fcn2 : TransferFcn  Denominator=[1 1.5]
  Transfer Fcn3 : TransferFcn  Denominator=[1 1.5]
  Out1 : Outport
  wires:
  Transfer Fcn2/1 -> Transfer Fcn3/1
  In1/1 -> Transfer Fcn2/1
  Transfer Fcn3/1 -> Out1/1

== system exp9_/Subsystem3/K = 7/K = 1/K = 1/K = 1 ==
  In1 : Inport
  Transfer Fcn2 : TransferFcn  Denominator=[1 1.5]
  Transfer Fcn3 : TransferFcn  Denominator=[1 1.5]
  Out1 : Outport
  wires:
  Transfer Fcn2/1 -> Transfer Fcn3/1
  In1/1 -> Transfer Fcn2/1
  Transfer Fcn3/1 -> Out1/1

== system exp9_/Subsystem3/K = 8/K = 1/K = 1/K = 1 ==
  In1 : Inport
  Transfer Fcn2 : TransferFcn  Denominator=[1 1.5]
  Transfer Fcn3 : TransferFcn  Denominator=[1 1.5]
  Out1 : Outport
  wires:
  Transfer Fcn2/1 -> Transfer Fcn3/1
  In1/1 -> Transfer Fcn2/1
  Transfer Fcn3/1 -> Out1/1

== system exp9_/Subsystem3/K = 9/K = 1/K = 1/K = 1 ==
  In1 : Inport
  Transfer Fcn2 : TransferFcn  Denominator=[1 1.5]
  Transfer Fcn3 : TransferFcn  Denominator=[1 1.5]
  Out1 : Outport
  wires:
  Transfer Fcn2/1 -> Transfer Fcn3/1
  In1/1 -> Transfer Fcn2/1
  Transfer Fcn3/1 -> Out1/1
